simulink model "ScriptDemo"  (R2022b)
settings: configuration reference "TmVcThermal_Configuration_sub" (kept outside this file)
undefined symbols (not defined in the file): aaaa, bbbb, cTmComprCtrl_D_u8HvacFlowTable_db, cTmComprCtrl_D_u8HvacFlowTable_sw, cTmComprCtrl_n_i16ChillCmpIMax, cTmComprCtrl_n_i16ChillCmpIMin, cTmComprCtrl_n_i16ChillCmpIMin666, cTmComprCtrl_n_i16ChillCmpPMax, cTmComprCtrl_n_i16ChillCmpPMin, cTmComprCtrl_n_i16CmpChillCoolRpmKiMax, cTmComprCtrl_n_i16CmpChillCoolRpmKiMin, cTmComprCtrl_n_i16CmpChillCoolRpmKpMax, cTmComprCtrl_n_i16CmpChillCoolRpmKpMin, cTmComprCtrl_n_i16CmpCoolRpmKiMax, cTmComprCtrl_n_i16CmpCoolRpmKiMin, cTmComprCtrl_n_i16CmpCoolRpmKpMax, cTmComprCtrl_n_i16CmpCoolRpmKpMin, cTmComprCtrl_n_i16SM4CmpHeatKiMax, cTmComprCtrl_n_i16SM4CmpHeatKiMin, cTmComprCtrl_n_i16SM4CmpHeatKpMax, cTmComprCtrl_n_i16SM4CmpHeatKpMin, cTmComprCtrl_n_i16SM5CmpHeatKiMax, cTmComprCtrl_n_i16SM5CmpHeatKiMin, cTmComprCtrl_n_i16SM5CmpHeatKpMax, cTmComprCtrl_n_i16SM5CmpHeatKpMin, cTmComprCtrl_n_i16SM6CmpHeatKiMax, cTmComprCtrl_n_i16SM6CmpHeatKiMin, cTmComprCtrl_n_i16SM6CmpHeatKpMax, cTmComprCtrl_n_i16SM6CmpHeatKpMin, cTmComprCtrl_n_u16CmpMaxSpdFanFltLimt, cTmComprCtrl_n_u16CmpMaxSpdLoSidePFltLimt, cTmComprCtrl_n_u16CmpMaxSpdSensorFltLimt, cTmComprCtrl_n_u16CompMinRpm, cTmComprCtrl_n_u16CompRpmIncThres, cTmComprCtrl_t_u16BattCooltFFPeriod, cTmComprCtrl_t_u16BattCooltPIPeriod, cTmComprCtrl_t_u16CmpCoolFFPeriod, cTmComprCtrl_t_u16CmpCoolPIPeriod, cTmComprCtrl_t_u16CoolCmpChillFFPeriod, cTmComprCtrl_t_u16CoolCmpChillPIPeriod, cTmComprCtrl_t_u16SM4CmpHeatFFPeriod, cTmComprCtrl_t_u16SM4CmpHeatPIPeriod, cTmComprCtrl_t_u16SM5CmpHeatFFPeriod, cTmComprCtrl_t_u16SM5CmpHeatPIPeriod, cTmComprCtrl_t_u16SM6CmpHeatFFPeriod, cTmComprCtrl_t_u16SM6CmpHeatPIPeriod, cTmComprCtrl_Te_EvapClearInteg, cTmComprCtrl_Te_i16HpReqTempSaturoffset, cTmComprCtrl_Te_i16SatLpReplaceDiff, cTmComprCtrl_Te_i16SM3BatDiffStartEvapDecOffset, cTmComprCtrl_Te_i16SM3EvapLo, cTmComprCtrl_Te_i16SM3TBatDiffEntEvapDecOffset, cTmComprCtrl_Te_i16SM3TBatDiffEntEvapDecOffsetQuit, cTmComprCtrl_Te_s32ErrCmpChillPIContinueCoolH, cTmComprCtrl_Te_s32ErrCmpChillPIContinueCoolL, cTmComprCtrl_Te_s32ErrCmpPIContinueChillH, cTmComprCtrl_Te_s32ErrCmpPIContinueChillL, cTmComprCtrl_Te_s32ErrCmpPIContinueCoolH, cTmComprCtrl_Te_s32ErrCmpPIContinueCoolL, cTmComprCtrl_Te_s32ErrCmpPIContinueHeatH ... (+398)
libraries: simulink x782, PCMULib x640, simulink_need_slupdate x4
(part 2 of 41)

== system ScriptDemo/Change/changeModSizeGcs/Before ==
  rTmComprCtrl_n_u16CompRpmReqModeOut : Inport  OutDataTypeStr=uint16
  sTmDiag_D_u8CmprDischrgTFltSt : Inport  Port=2  OutDataTypeStr=uint8
  sTmDiag_D_u8FanFltSt : Inport  Port=3  OutDataTypeStr=uint8
  sTmDiag_D_u8HiSidePFltSt : Inport  Port=4  OutDataTypeStr=uint8
  sTmDiag_D_u8OutrCondOutTFltSt : Inport  Port=5  OutDataTypeStr=uint8
  sTmSigProces_Te_s32TAmb : Inport  Port=6  OutDataTypeStr=single
  sTmIn_n_s32ElacCmprActl : Inport  Port=7  OutDataTypeStr=single
  sTmIn_v_s32VehSpdLgt : Inport  Port=8  OutDataTypeStr=single
  sTmRefriModeMgr_D_u8HPCurMode : Inport  Port=9  OutDataTypeStr=uint8
  sTmRefriModeMgr_D_u8HpFmCmd : Inport  Port=10  OutDataTypeStr=uint8
  sTmSigProces_Pw_i16ReqPwrForHeat : Inport  Port=11  OutDataTypeStr=int16
  sTmSigProces_Te_s32CompDischarge : Inport  Port=12  OutDataTypeStr=single
  sTmSigProces_md_u16BlwCool : Inport  Port=13  OutDataTypeStr=uint16
  sTmSigProces_p_u16PHighSide : Inport  Port=14  OutDataTypeStr=uint16
  sTmSigProces_p_u16PLowSide : Inport  Port=15  OutDataTypeStr=uint16
  sTmIn_D_u8HeatPump : Inport  Port=16  OutDataTypeStr=uint8
  sTmIn_D_u8ElecDriveline : Inport  Port=17
  sTmSigProces_D_u8CarChrgMode : Inport  Port=18  OutDataTypeStr=uint8
  sTmSigProces_md_u16BlwHeat : Inport  Port=19  OutDataTypeStr=uint16
  sTmDiag_D_u8LoSidePFltSt : Inport  Port=20  OutDataTypeStr=uint8
  xTmComprCtrl_B_CompOnReqCompOn : Inport  Port=21  OutDataTypeStr=boolean
  rTmComprCtrl_n_u16CompRpmReqModeOut1 : Inport  Port=22  OutDataTypeStr=uint16
  sTmDiag_D_u8CmprDischrgTFltSt1 : Inport  Port=23  OutDataTypeStr=uint8
  sTmDiag_D_u8FanFltSt1 : Inport  Port=24  OutDataTypeStr=uint8
  sTmDiag_D_u8HiSidePFltSt1 : Inport  Port=25  OutDataTypeStr=uint8
  sTmDiag_D_u8OutrCondOutTFltSt1 : Inport  Port=26  OutDataTypeStr=uint8
  sTmSigProces_Te_s32TAmb1 : Inport  Port=27  OutDataTypeStr=single
  sTmIn_n_s32ElacCmprActl1 : Inport  Port=28  OutDataTypeStr=single
  sTmIn_v_s32VehSpdLgt1 : Inport  Port=29  OutDataTypeStr=single
  sTmRefriModeMgr_D_u8HPCurMode1 : Inport  Port=30  OutDataTypeStr=uint8
  sTmRefriModeMgr_D_u8HpFmCmd1 : Inport  Port=31  OutDataTypeStr=uint8
  sTmSigProces_Pw_i16ReqPwrForHeat1 : Inport  Port=32  OutDataTypeStr=int16
  sTmSigProces_Te_s32CompDischarge1 : Inport  Port=33  OutDataTypeStr=single
  rTmComprCtrl_n_u16CompRpmReqModeOut2 : Inport  Port=34  OutDataTypeStr=uint16
  sTmDiag_D_u8CmprDischrgTFltSt2 : Inport  Port=35  OutDataTypeStr=uint8
  sTmDiag_D_u8FanFltSt2 : Inport  Port=36  OutDataTypeStr=uint8
  sTmDiag_D_u8HiSidePFltSt2 : Inport  Port=37  OutDataTypeStr=uint8
  sTmDiag_D_u8OutrCondOutTFltSt2 : Inport  Port=38  OutDataTypeStr=uint8
  sTmSigProces_Te_s32TAmb2 : Inport  Port=39  OutDataTypeStr=single
  sTmIn_n_s32ElacCmprActl2 : Inport  Port=40  OutDataTypeStr=single
  sTmIn_v_s32VehSpdLgt2 : Inport  Port=41  OutDataTypeStr=single
  sTmRefriModeMgr_D_u8HPCurMode2 : Inport  Port=42  OutDataTypeStr=uint8
  sTmRefriModeMgr_D_u8HpFmCmd2 : Inport  Port=43  OutDataTypeStr=uint8
  sTmSigProces_Pw_i16ReqPwrForHeat2 : Inport  Port=44  OutDataTypeStr=int16
  sTmSigProces_Te_s32CompDischarge2 : Inport  Port=45  OutDataTypeStr=single
  sTmSigProces_md_u16BlwCool2 : Inport  Port=46  OutDataTypeStr=uint16
  sTmSigProces_p_u16PHighSide2 : Inport  Port=47  OutDataTypeStr=uint16
  sTmSigProces_p_u16PLowSide2 : Inport  Port=48  OutDataTypeStr=uint16
  sTmIn_D_u8HeatPump2 : Inport  Port=49  OutDataTypeStr=uint8
  sTmIn_D_u8ElecDriveline2 : Inport  Port=50
  sTmSigProces_D_u8CarChrgMode2 : Inport  Port=51  OutDataTypeStr=uint8
  sTmSigProces_md_u16BlwHeat2 : Inport  Port=52  OutDataTypeStr=uint16
  sTmDiag_D_u8LoSidePFltSt2 : Inport  Port=53  OutDataTypeStr=uint8
  xTmComprCtrl_B_CompOnReqCompOn2 : Inport  Port=54  OutDataTypeStr=boolean
  rTmComprCtrl_n_u16CompRpmReqModeOut3 : Inport  Port=55  OutDataTypeStr=uint16
  sTmDiag_D_u8CmprDischrgTFltSt3 : Inport  Port=56  OutDataTypeStr=uint8
  sTmDiag_D_u8FanFltSt3 : Inport  Port=57  OutDataTypeStr=uint8
  sTmDiag_D_u8HiSidePFltSt3 : Inport  Port=58  OutDataTypeStr=uint8
  sTmDiag_D_u8OutrCondOutTFltSt3 : Inport  Port=59  OutDataTypeStr=uint8
  sTmSigProces_Te_s32TAmb3 : Inport  Port=60  OutDataTypeStr=single
  sTmIn_n_s32ElacCmprActl3 : Inport  Port=61  OutDataTypeStr=single
  sTmIn_v_s32VehSpdLgt3 : Inport  Port=62  OutDataTypeStr=single
  sTmRefriModeMgr_D_u8HPCurMode3 : Inport  Port=63  OutDataTypeStr=uint8
  sTmRefriModeMgr_D_u8HpFmCmd3 : Inport  Port=64  OutDataTypeStr=uint8
  sTmSigProces_Pw_i16ReqPwrForHeat3 : Inport  Port=65  OutDataTypeStr=int16
  sTmSigProces_Te_s32CompDischarge3 : Inport  Port=66  OutDataTypeStr=single
  sTmSigProces_md_u16BlwCool3 : Inport  Port=67  OutDataTypeStr=uint16
  sTmSigProces_p_u16PHighSide3 : Inport  Port=68  OutDataTypeStr=uint16
  sTmSigProces_p_u16PLowSide3 : Inport  Port=69  OutDataTypeStr=uint16
  sTmIn_D_u8HeatPump3 : Inport  Port=70  OutDataTypeStr=uint8
  sTmIn_D_u8ElecDriveline3 : Inport  Port=71
  sTmSigProces_D_u8CarChrgMode3 : Inport  Port=72  OutDataTypeStr=uint8
  sTmSigProces_md_u16BlwHeat3 : Inport  Port=73  OutDataTypeStr=uint16
  sTmDiag_D_u8LoSidePFltSt3 : Inport  Port=74  OutDataTypeStr=uint8
  xTmComprCtrl_B_CompOnReqCompOn3 : Inport  Port=75  OutDataTypeStr=boolean
  Subsystem : Subsystem
  Subsystem1 : Subsystem
  Subsystem2 : Subsystem
  Subsystem3 : Subsystem
  rTmComprCtrl_n_u16CompRpmReqFilter : Outport  OutDataTypeStr=uint16
  xTmComprCtrl_B_KeepRpm : Outport  Port=2  OutDataTypeStr=boolean
  xFilter_B_ComprStop : Outport  Port=3  OutDataTypeStr=boolean
  sFilter_n_u16CompMaxRpm : Outport  Port=4  OutDataTypeStr=uint16
  rFilter_p_u16AcHiSideHiCut : Outport  Port=5  OutDataTypeStr=uint16
  rFilter_p_u16CmpLimitNormalP : Outport  Port=6  OutDataTypeStr=uint16
  rFilter_p_u16CmpLimitLowP : Outport  Port=7  OutDataTypeStr=uint16
  rFilter_p_u16CmpLimitMidP : Outport  Port=8  OutDataTypeStr=uint16
  rFilter_p_u16CmpLimitShutDownP : Outport  Port=9  OutDataTypeStr=uint16
  xTmComprCtrl_B_ReduceRpm : Outport  Port=10  OutDataTypeStr=boolean
  rTmComprCtrl_n_u16CompRpmReqFilter1 : Outport  Port=11  OutDataTypeStr=uint16
  xTmComprCtrl_B_KeepRpm1 : Outport  Port=12  OutDataTypeStr=boolean
  xFilter_B_ComprStop1 : Outport  Port=13  OutDataTypeStr=boolean
  sFilter_n_u16CompMaxRpm1 : Outport  Port=14  OutDataTypeStr=uint16
  rFilter_p_u16AcHiSideHiCut1 : Outport  Port=15  OutDataTypeStr=uint16
  rFilter_p_u16CmpLimitNormalP1 : Outport  Port=16  OutDataTypeStr=uint16
  rFilter_p_u16CmpLimitLowP1 : Outport  Port=17  OutDataTypeStr=uint16
  rFilter_p_u16CmpLimitMidP1 : Outport  Port=18  OutDataTypeStr=uint16
  rFilter_p_u16CmpLimitShutDownP1 : Outport  Port=19  OutDataTypeStr=uint16
  xTmComprCtrl_B_ReduceRpm1 : Outport  Port=20  OutDataTypeStr=boolean
  rTmComprCtrl_n_u16CompRpmReqFilter2 : Outport  Port=21  OutDataTypeStr=uint16
  xTmComprCtrl_B_KeepRpm2 : Outport  Port=22  OutDataTypeStr=boolean
  xFilter_B_ComprStop2 : Outport  Port=23  OutDataTypeStr=boolean
  sFilter_n_u16CompMaxRpm2 : Outport  Port=24  OutDataTypeStr=uint16
  rFilter_p_u16AcHiSideHiCut2 : Outport  Port=25  OutDataTypeStr=uint16
  rFilter_p_u16CmpLimitNormalP2 : Outport  Port=26  OutDataTypeStr=uint16
  rFilter_p_u16CmpLimitLowP2 : Outport  Port=27  OutDataTypeStr=uint16
  rFilter_p_u16CmpLimitMidP2 : Outport  Port=28  OutDataTypeStr=uint16
  rFilter_p_u16CmpLimitShutDownP2 : Outport  Port=29  OutDataTypeStr=uint16
  xTmComprCtrl_B_ReduceRpm2 : Outport  Port=30  OutDataTypeStr=boolean
  rTmComprCtrl_n_u16CompRpmReqFilter3 : Outport  Port=31  OutDataTypeStr=uint16
  xTmComprCtrl_B_KeepRpm3 : Outport  Port=32  OutDataTypeStr=boolean
  xFilter_B_ComprStop3 : Outport  Port=33  OutDataTypeStr=boolean
  sFilter_n_u16CompMaxRpm3 : Outport  Port=34  OutDataTypeStr=uint16
  rFilter_p_u16AcHiSideHiCut3 : Outport  Port=35  OutDataTypeStr=uint16
  rFilter_p_u16CmpLimitNormalP3 : Outport  Port=36  OutDataTypeStr=uint16
  rFilter_p_u16CmpLimitLowP3 : Outport  Port=37  OutDataTypeStr=uint16
  rFilter_p_u16CmpLimitMidP3 : Outport  Port=38  OutDataTypeStr=uint16
  rFilter_p_u16CmpLimitShutDownP3 : Outport  Port=39  OutDataTypeStr=uint16
  xTmComprCtrl_B_ReduceRpm3 : Outport  Port=40  OutDataTypeStr=boolean
  wires:
  Subsystem/7(rFilter_p_u16CmpLimitLowP) -> rFilter_p_u16CmpLimitLowP/1
  Subsystem/2(xTmComprCtrl_B_KeepRpm) -> xTmComprCtrl_B_KeepRpm/1
  Subsystem/8(rFilter_p_u16CmpLimitMidP) -> rFilter_p_u16CmpLimitMidP/1
  Subsystem/9(rFilter_p_u16CmpLimitShutDownP) -> rFilter_p_u16CmpLimitShutDownP/1
  Subsystem/6(rFilter_p_u16CmpLimitNormalP) -> rFilter_p_u16CmpLimitNormalP/1
  Subsystem/5(rFilter_p_u16AcHiSideHiCut) -> rFilter_p_u16AcHiSideHiCut/1
  Subsystem/3(xFilter_B_ComprStop) -> xFilter_B_ComprStop/1
  Subsystem/4(sFilter_n_u16CompMaxRpm) -> sFilter_n_u16CompMaxRpm/1
  sTmSigProces_D_u8CarChrgMode/1 -> Subsystem/18(sTmSigProces_D_u8CarChrgMode)
  sTmSigProces_md_u16BlwHeat/1 -> Subsystem/19(sTmSigProces_md_u16BlwHeat)
  sTmSigProces_p_u16PLowSide/1 -> Subsystem/15(sTmSigProces_p_u16PLowSide)
  sTmIn_D_u8HeatPump/1 -> Subsystem/16(sTmIn_D_u8HeatPump)
  sTmIn_D_u8ElecDriveline/1 -> Subsystem/17(sTmIn_D_u8ElecDriveline)
  sTmDiag_D_u8LoSidePFltSt/1 -> Subsystem/20(sTmDiag_D_u8LoSidePFltSt)
  sTmSigProces_Te_s32TAmb/1 -> Subsystem/6(sTmSigProces_Te_s32TAmb)
  sTmIn_n_s32ElacCmprActl/1 -> Subsystem/7(sTmIn_n_s32ElacCmprActl)
  sTmSigProces_Te_s32CompDischarge/1 -> Subsystem/12(sTmSigProces_Te_s32CompDischarge)
  sTmRefriModeMgr_D_u8HPCurMode/1 -> Subsystem/9(sTmRefriModeMgr_D_u8HPCurMode)
  sTmSigProces_Pw_i16ReqPwrForHeat/1 -> Subsystem/11(sTmSigProces_Pw_i16ReqPwrForHeat)
  sTmRefriModeMgr_D_u8HpFmCmd/1 -> Subsystem/10(sTmRefriModeMgr_D_u8HpFmCmd)
  sTmDiag_D_u8OutrCondOutTFltSt/1 -> Subsystem/5(sTmDiag_D_u8OutrCondOutTFltSt)
  sTmIn_v_s32VehSpdLgt/1 -> Subsystem/8(sTmIn_v_s32VehSpdLgt)
  sTmSigProces_md_u16BlwCool/1 -> Subsystem/13(sTmSigProces_md_u16BlwCool)
  sTmDiag_D_u8FanFltSt/1 -> Subsystem/3(sTmDiag_D_u8FanFltSt)
  sTmDiag_D_u8HiSidePFltSt/1 -> Subsystem/4(sTmDiag_D_u8HiSidePFltSt)
  xTmComprCtrl_B_CompOnReqCompOn/1 -> Subsystem/21(xTmComprCtrl_B_CompOnReqCompOn)
  sTmDiag_D_u8CmprDischrgTFltSt/1 -> Subsystem/2(sTmDiag_D_u8CmprDischrgTFltSt)
  rTmComprCtrl_n_u16CompRpmReqModeOut/1 -> Subsystem/1(rTmComprCtrl_n_u16CompRpmReqModeOut)
  Subsystem/1(rTmComprCtrl_n_u16CompRpmReqFilter) -> rTmComprCtrl_n_u16CompRpmReqFilter/1
  sTmSigProces_p_u16PHighSide/1 -> Subsystem/14(sTmSigProces_p_u16PHighSide)
  Subsystem/10(xTmComprCtrl_B_ReduceRpm) -> xTmComprCtrl_B_ReduceRpm/1
  Subsystem1/1(rTmComprCtrl_n_u16CompRpmReqFilter) -> rTmComprCtrl_n_u16CompRpmReqFilter1/1
  Subsystem1/10(xTmComprCtrl_B_ReduceRpm) -> xTmComprCtrl_B_ReduceRpm1/1
  rTmComprCtrl_n_u16CompRpmReqModeOut1/1 -> Subsystem1/1(rTmComprCtrl_n_u16CompRpmReqModeOut)
  sTmDiag_D_u8HiSidePFltSt1/1 -> Subsystem1/4(sTmDiag_D_u8HiSidePFltSt)
  sTmDiag_D_u8FanFltSt1/1 -> Subsystem1/3(sTmDiag_D_u8FanFltSt)
  Subsystem1/2(xTmComprCtrl_B_KeepRpm) -> xTmComprCtrl_B_KeepRpm1/1
  Subsystem1/7(rFilter_p_u16CmpLimitLowP) -> rFilter_p_u16CmpLimitLowP1/1
  sTmDiag_D_u8OutrCondOutTFltSt1/1 -> Subsystem1/5(sTmDiag_D_u8OutrCondOutTFltSt)
  sTmSigProces_Pw_i16ReqPwrForHeat1/1 -> Subsystem1/11(sTmSigProces_Pw_i16ReqPwrForHeat)
  sTmRefriModeMgr_D_u8HpFmCmd1/1 -> Subsystem1/10(sTmRefriModeMgr_D_u8HpFmCmd)
  sTmSigProces_Te_s32CompDischarge1/1 -> Subsystem1/12(sTmSigProces_Te_s32CompDischarge)
  sTmIn_n_s32ElacCmprActl1/1 -> Subsystem1/7(sTmIn_n_s32ElacCmprActl)
  sTmRefriModeMgr_D_u8HPCurMode1/1 -> Subsystem1/9(sTmRefriModeMgr_D_u8HPCurMode)
  sTmIn_v_s32VehSpdLgt1/1 -> Subsystem1/8(sTmIn_v_s32VehSpdLgt)
  Subsystem1/3(xFilter_B_ComprStop) -> xFilter_B_ComprStop1/1
  sTmSigProces_Te_s32TAmb1/1 -> Subsystem1/6(sTmSigProces_Te_s32TAmb)
  Subsystem1/5(rFilter_p_u16AcHiSideHiCut) -> rFilter_p_u16AcHiSideHiCut1/1
  sTmDiag_D_u8CmprDischrgTFltSt1/1 -> Subsystem1/2(sTmDiag_D_u8CmprDischrgTFltSt)
  Subsystem1/6(rFilter_p_u16CmpLimitNormalP) -> rFilter_p_u16CmpLimitNormalP1/1
  Subsystem1/4(sFilter_n_u16CompMaxRpm) -> sFilter_n_u16CompMaxRpm1/1
  Subsystem1/9(rFilter_p_u16CmpLimitShutDownP) -> rFilter_p_u16CmpLimitShutDownP1/1
  Subsystem1/8(rFilter_p_u16CmpLimitMidP) -> rFilter_p_u16CmpLimitMidP1/1
  Subsystem2/1(rTmComprCtrl_n_u16CompRpmReqFilter) -> rTmComprCtrl_n_u16CompRpmReqFilter2/1
  Subsystem2/10(xTmComprCtrl_B_ReduceRpm) -> xTmComprCtrl_B_ReduceRpm2/1
  sTmSigProces_p_u16PHighSide2/1 -> Subsystem2/14(sTmSigProces_p_u16PHighSide)
  rTmComprCtrl_n_u16CompRpmReqModeOut2/1 -> Subsystem2/1(rTmComprCtrl_n_u16CompRpmReqModeOut)
  sTmDiag_D_u8HiSidePFltSt2/1 -> Subsystem2/4(sTmDiag_D_u8HiSidePFltSt)
  sTmDiag_D_u8FanFltSt2/1 -> Subsystem2/3(sTmDiag_D_u8FanFltSt)
  Subsystem2/2(xTmComprCtrl_B_KeepRpm) -> xTmComprCtrl_B_KeepRpm2/1
  Subsystem2/7(rFilter_p_u16CmpLimitLowP) -> rFilter_p_u16CmpLimitLowP2/1
  sTmSigProces_md_u16BlwCool2/1 -> Subsystem2/13(sTmSigProces_md_u16BlwCool)
  sTmDiag_D_u8LoSidePFltSt2/1 -> Subsystem2/20(sTmDiag_D_u8LoSidePFltSt)
  sTmDiag_D_u8OutrCondOutTFltSt2/1 -> Subsystem2/5(sTmDiag_D_u8OutrCondOutTFltSt)
  xTmComprCtrl_B_CompOnReqCompOn2/1 -> Subsystem2/21(xTmComprCtrl_B_CompOnReqCompOn)
  sTmSigProces_Pw_i16ReqPwrForHeat2/1 -> Subsystem2/11(sTmSigProces_Pw_i16ReqPwrForHeat)
  sTmRefriModeMgr_D_u8HpFmCmd2/1 -> Subsystem2/10(sTmRefriModeMgr_D_u8HpFmCmd)
  sTmSigProces_Te_s32CompDischarge2/1 -> Subsystem2/12(sTmSigProces_Te_s32CompDischarge)
  sTmIn_n_s32ElacCmprActl2/1 -> Subsystem2/7(sTmIn_n_s32ElacCmprActl)
  sTmIn_D_u8HeatPump2/1 -> Subsystem2/16(sTmIn_D_u8HeatPump)
  sTmSigProces_p_u16PLowSide2/1 -> Subsystem2/15(sTmSigProces_p_u16PLowSide)
  sTmRefriModeMgr_D_u8HPCurMode2/1 -> Subsystem2/9(sTmRefriModeMgr_D_u8HPCurMode)
  sTmIn_v_s32VehSpdLgt2/1 -> Subsystem2/8(sTmIn_v_s32VehSpdLgt)
  sTmSigProces_D_u8CarChrgMode2/1 -> Subsystem2/18(sTmSigProces_D_u8CarChrgMode)
  Subsystem2/3(xFilter_B_ComprStop) -> xFilter_B_ComprStop2/1
  sTmSigProces_Te_s32TAmb2/1 -> Subsystem2/6(sTmSigProces_Te_s32TAmb)
  sTmSigProces_md_u16BlwHeat2/1 -> Subsystem2/19(sTmSigProces_md_u16BlwHeat)
  Subsystem2/5(rFilter_p_u16AcHiSideHiCut) -> rFilter_p_u16AcHiSideHiCut2/1
  sTmDiag_D_u8CmprDischrgTFltSt2/1 -> Subsystem2/2(sTmDiag_D_u8CmprDischrgTFltSt)
  Subsystem2/6(rFilter_p_u16CmpLimitNormalP) -> rFilter_p_u16CmpLimitNormalP2/1
  Subsystem2/4(sFilter_n_u16CompMaxRpm) -> sFilter_n_u16CompMaxRpm2/1
  sTmIn_D_u8ElecDriveline2/1 -> Subsystem2/17(sTmIn_D_u8ElecDriveline)
  Subsystem2/9(rFilter_p_u16CmpLimitShutDownP) -> rFilter_p_u16CmpLimitShutDownP2/1
  Subsystem2/8(rFilter_p_u16CmpLimitMidP) -> rFilter_p_u16CmpLimitMidP2/1
  Subsystem3/1(rTmComprCtrl_n_u16CompRpmReqFilter) -> rTmComprCtrl_n_u16CompRpmReqFilter3/1
  Subsystem3/10(xTmComprCtrl_B_ReduceRpm) -> xTmComprCtrl_B_ReduceRpm3/1
  sTmSigProces_p_u16PHighSide3/1 -> Subsystem3/14(sTmSigProces_p_u16PHighSide)
  rTmComprCtrl_n_u16CompRpmReqModeOut3/1 -> Subsystem3/1(rTmComprCtrl_n_u16CompRpmReqModeOut)
  sTmDiag_D_u8HiSidePFltSt3/1 -> Subsystem3/4(sTmDiag_D_u8HiSidePFltSt)
  sTmDiag_D_u8FanFltSt3/1 -> Subsystem3/3(sTmDiag_D_u8FanFltSt)
  Subsystem3/2(xTmComprCtrl_B_KeepRpm) -> xTmComprCtrl_B_KeepRpm3/1
  Subsystem3/7(rFilter_p_u16CmpLimitLowP) -> rFilter_p_u16CmpLimitLowP3/1
  sTmSigProces_md_u16BlwCool3/1 -> Subsystem3/13(sTmSigProces_md_u16BlwCool)
  sTmDiag_D_u8LoSidePFltSt3/1 -> Subsystem3/20(sTmDiag_D_u8LoSidePFltSt)
  sTmDiag_D_u8OutrCondOutTFltSt3/1 -> Subsystem3/5(sTmDiag_D_u8OutrCondOutTFltSt)
  xTmComprCtrl_B_CompOnReqCompOn3/1 -> Subsystem3/21(xTmComprCtrl_B_CompOnReqCompOn)
  sTmSigProces_Pw_i16ReqPwrForHeat3/1 -> Subsystem3/11(sTmSigProces_Pw_i16ReqPwrForHeat)
  sTmRefriModeMgr_D_u8HpFmCmd3/1 -> Subsystem3/10(sTmRefriModeMgr_D_u8HpFmCmd)
  sTmSigProces_Te_s32CompDischarge3/1 -> Subsystem3/12(sTmSigProces_Te_s32CompDischarge)
  sTmIn_n_s32ElacCmprActl3/1 -> Subsystem3/7(sTmIn_n_s32ElacCmprActl)
  sTmIn_D_u8HeatPump3/1 -> Subsystem3/16(sTmIn_D_u8HeatPump)
  sTmSigProces_p_u16PLowSide3/1 -> Subsystem3/15(sTmSigProces_p_u16PLowSide)
  sTmRefriModeMgr_D_u8HPCurMode3/1 -> Subsystem3/9(sTmRefriModeMgr_D_u8HPCurMode)
  sTmIn_v_s32VehSpdLgt3/1 -> Subsystem3/8(sTmIn_v_s32VehSpdLgt)
  sTmSigProces_D_u8CarChrgMode3/1 -> Subsystem3/18(sTmSigProces_D_u8CarChrgMode)
  Subsystem3/3(xFilter_B_ComprStop) -> xFilter_B_ComprStop3/1
  sTmSigProces_Te_s32TAmb3/1 -> Subsystem3/6(sTmSigProces_Te_s32TAmb)
  sTmSigProces_md_u16BlwHeat3/1 -> Subsystem3/19(sTmSigProces_md_u16BlwHeat)
  Subsystem3/5(rFilter_p_u16AcHiSideHiCut) -> rFilter_p_u16AcHiSideHiCut3/1
  sTmDiag_D_u8CmprDischrgTFltSt3/1 -> Subsystem3/2(sTmDiag_D_u8CmprDischrgTFltSt)
  Subsystem3/6(rFilter_p_u16CmpLimitNormalP) -> rFilter_p_u16CmpLimitNormalP3/1
  Subsystem3/4(sFilter_n_u16CompMaxRpm) -> sFilter_n_u16CompMaxRpm3/1
  sTmIn_D_u8ElecDriveline3/1 -> Subsystem3/17(sTmIn_D_u8ElecDriveline)
  Subsystem3/9(rFilter_p_u16CmpLimitShutDownP) -> rFilter_p_u16CmpLimitShutDownP3/1
  Subsystem3/8(rFilter_p_u16CmpLimitMidP) -> rFilter_p_u16CmpLimitMidP3/1

== system ScriptDemo/Change/changeModSizeGcs/Before1 ==
  rTmComprCtrl_n_u16CompRpmReqModeOut : Inport  OutDataTypeStr=uint16
  sTmDiag_D_u8CmprDischrgTFltSt : Inport  Port=2  OutDataTypeStr=uint8
  sTmDiag_D_u8FanFltSt : Inport  Port=3  OutDataTypeStr=uint8
  sTmDiag_D_u8HiSidePFltSt : Inport  Port=4  OutDataTypeStr=uint8
  sTmDiag_D_u8OutrCondOutTFltSt : Inport  Port=5  OutDataTypeStr=uint8
  sTmSigProces_Te_s32TAmb : Inport  Port=6  OutDataTypeStr=single
  sTmIn_n_s32ElacCmprActl : Inport  Port=7  OutDataTypeStr=single
  sTmIn_v_s32VehSpdLgt : Inport  Port=8  OutDataTypeStr=single
  sTmRefriModeMgr_D_u8HPCurMode : Inport  Port=9  OutDataTypeStr=uint8
  sTmRefriModeMgr_D_u8HpFmCmd : Inport  Port=10  OutDataTypeStr=uint8
  sTmSigProces_Pw_i16ReqPwrForHeat : Inport  Port=11  OutDataTypeStr=int16
  sTmSigProces_Te_s32CompDischarge : Inport  Port=12  OutDataTypeStr=single
  sTmSigProces_md_u16BlwCool : Inport  Port=13  OutDataTypeStr=uint16
  sTmSigProces_p_u16PHighSide : Inport  Port=14  OutDataTypeStr=uint16
  sTmSigProces_p_u16PLowSide : Inport  Port=15  OutDataTypeStr=uint16
  sTmIn_D_u8HeatPump : Inport  Port=16  OutDataTypeStr=uint8
  sTmIn_D_u8ElecDriveline : Inport  Port=17
  sTmSigProces_D_u8CarChrgMode : Inport  Port=18  OutDataTypeStr=uint8
  sTmSigProces_md_u16BlwHeat : Inport  Port=19  OutDataTypeStr=uint16
  sTmDiag_D_u8LoSidePFltSt : Inport  Port=20  OutDataTypeStr=uint8
  xTmComprCtrl_B_CompOnReqCompOn : Inport  Port=21  OutDataTypeStr=boolean
  rTmComprCtrl_n_u16CompRpmReqModeOut1 : Inport  Port=22  OutDataTypeStr=uint16
  sTmDiag_D_u8CmprDischrgTFltSt1 : Inport  Port=23  OutDataTypeStr=uint8
  sTmDiag_D_u8FanFltSt1 : Inport  Port=24  OutDataTypeStr=uint8
  sTmDiag_D_u8HiSidePFltSt1 : Inport  Port=25  OutDataTypeStr=uint8
  sTmDiag_D_u8OutrCondOutTFltSt1 : Inport  Port=26  OutDataTypeStr=uint8
  sTmSigProces_Te_s32TAmb1 : Inport  Port=27  OutDataTypeStr=single
  sTmIn_n_s32ElacCmprActl1 : Inport  Port=28  OutDataTypeStr=single
  sTmIn_v_s32VehSpdLgt1 : Inport  Port=29  OutDataTypeStr=single
  sTmRefriModeMgr_D_u8HPCurMode1 : Inport  Port=30  OutDataTypeStr=uint8
  sTmRefriModeMgr_D_u8HpFmCmd1 : Inport  Port=31  OutDataTypeStr=uint8
  sTmSigProces_Pw_i16ReqPwrForHeat1 : Inport  Port=32  OutDataTypeStr=int16
  sTmSigProces_Te_s32CompDischarge1 : Inport  Port=33  OutDataTypeStr=single
  rTmComprCtrl_n_u16CompRpmReqModeOut2 : Inport  Port=34  OutDataTypeStr=uint16
  sTmDiag_D_u8CmprDischrgTFltSt2 : Inport  Port=35  OutDataTypeStr=uint8
  sTmDiag_D_u8FanFltSt2 : Inport  Port=36  OutDataTypeStr=uint8
  sTmDiag_D_u8HiSidePFltSt2 : Inport  Port=37  OutDataTypeStr=uint8
  sTmDiag_D_u8OutrCondOutTFltSt2 : Inport  Port=38  OutDataTypeStr=uint8
  sTmSigProces_Te_s32TAmb2 : Inport  Port=39  OutDataTypeStr=single
  sTmIn_n_s32ElacCmprActl2 : Inport  Port=40  OutDataTypeStr=single
  sTmIn_v_s32VehSpdLgt2 : Inport  Port=41  OutDataTypeStr=single
  sTmRefriModeMgr_D_u8HPCurMode2 : Inport  Port=42  OutDataTypeStr=uint8
  sTmRefriModeMgr_D_u8HpFmCmd2 : Inport  Port=43  OutDataTypeStr=uint8
  sTmSigProces_Pw_i16ReqPwrForHeat2 : Inport  Port=44  OutDataTypeStr=int16
  sTmSigProces_Te_s32CompDischarge2 : Inport  Port=45  OutDataTypeStr=single
  sTmSigProces_md_u16BlwCool2 : Inport  Port=46  OutDataTypeStr=uint16
  sTmSigProces_p_u16PHighSide2 : Inport  Port=47  OutDataTypeStr=uint16
  sTmSigProces_p_u16PLowSide2 : Inport  Port=48  OutDataTypeStr=uint16
  sTmIn_D_u8HeatPump2 : Inport  Port=49  OutDataTypeStr=uint8
  sTmIn_D_u8ElecDriveline2 : Inport  Port=50
  sTmSigProces_D_u8CarChrgMode2 : Inport  Port=51  OutDataTypeStr=uint8
  sTmSigProces_md_u16BlwHeat2 : Inport  Port=52  OutDataTypeStr=uint16
  sTmDiag_D_u8LoSidePFltSt2 : Inport  Port=53  OutDataTypeStr=uint8
  xTmComprCtrl_B_CompOnReqCompOn2 : Inport  Port=54  OutDataTypeStr=boolean
  rTmComprCtrl_n_u16CompRpmReqModeOut3 : Inport  Port=55  OutDataTypeStr=uint16
  sTmDiag_D_u8CmprDischrgTFltSt3 : Inport  Port=56  OutDataTypeStr=uint8
  sTmDiag_D_u8FanFltSt3 : Inport  Port=57  OutDataTypeStr=uint8
  sTmDiag_D_u8HiSidePFltSt3 : Inport  Port=58  OutDataTypeStr=uint8
  sTmDiag_D_u8OutrCondOutTFltSt3 : Inport  Port=59  OutDataTypeStr=uint8
  sTmSigProces_Te_s32TAmb3 : Inport  Port=60  OutDataTypeStr=single
  sTmIn_n_s32ElacCmprActl3 : Inport  Port=61  OutDataTypeStr=single
  sTmIn_v_s32VehSpdLgt3 : Inport  Port=62  OutDataTypeStr=single
  sTmRefriModeMgr_D_u8HPCurMode3 : Inport  Port=63  OutDataTypeStr=uint8
  sTmRefriModeMgr_D_u8HpFmCmd3 : Inport  Port=64  OutDataTypeStr=uint8
  sTmSigProces_Pw_i16ReqPwrForHeat3 : Inport  Port=65  OutDataTypeStr=int16
  sTmSigProces_Te_s32CompDischarge3 : Inport  Port=66  OutDataTypeStr=single
  sTmSigProces_md_u16BlwCool3 : Inport  Port=67  OutDataTypeStr=uint16
  sTmSigProces_p_u16PHighSide3 : Inport  Port=68  OutDataTypeStr=uint16
  sTmSigProces_p_u16PLowSide3 : Inport  Port=69  OutDataTypeStr=uint16
  sTmIn_D_u8HeatPump3 : Inport  Port=70  OutDataTypeStr=uint8
  sTmIn_D_u8ElecDriveline3 : Inport  Port=71
  sTmSigProces_D_u8CarChrgMode3 : Inport  Port=72  OutDataTypeStr=uint8
  sTmSigProces_md_u16BlwHeat3 : Inport  Port=73  OutDataTypeStr=uint16
  sTmDiag_D_u8LoSidePFltSt3 : Inport  Port=74  OutDataTypeStr=uint8
  xTmComprCtrl_B_CompOnReqCompOn3 : Inport  Port=75  OutDataTypeStr=boolean
  Subsystem : Subsystem
  Subsystem1 : Subsystem
  Subsystem2 : Subsystem
  Subsystem3 : Subsystem
  rTmComprCtrl_n_u16CompRpmReqFilter : Outport  OutDataTypeStr=uint16
  xTmComprCtrl_B_KeepRpm : Outport  Port=2  OutDataTypeStr=boolean
  xFilter_B_ComprStop : Outport  Port=3  OutDataTypeStr=boolean
  sFilter_n_u16CompMaxRpm : Outport  Port=4  OutDataTypeStr=uint16
  rFilter_p_u16AcHiSideHiCut : Outport  Port=5  OutDataTypeStr=uint16
  rFilter_p_u16CmpLimitNormalP : Outport  Port=6  OutDataTypeStr=uint16
  rFilter_p_u16CmpLimitLowP : Outport  Port=7  OutDataTypeStr=uint16
  rFilter_p_u16CmpLimitMidP : Outport  Port=8  OutDataTypeStr=uint16
  rFilter_p_u16CmpLimitShutDownP : Outport  Port=9  OutDataTypeStr=uint16
  xTmComprCtrl_B_ReduceRpm : Outport  Port=10  OutDataTypeStr=boolean
  rTmComprCtrl_n_u16CompRpmReqFilter1 : Outport  Port=11  OutDataTypeStr=uint16
  xTmComprCtrl_B_KeepRpm1 : Outport  Port=12  OutDataTypeStr=boolean
  xFilter_B_ComprStop1 : Outport  Port=13  OutDataTypeStr=boolean
  sFilter_n_u16CompMaxRpm1 : Outport  Port=14  OutDataTypeStr=uint16
  rFilter_p_u16AcHiSideHiCut1 : Outport  Port=15  OutDataTypeStr=uint16
  rFilter_p_u16CmpLimitNormalP1 : Outport  Port=16  OutDataTypeStr=uint16
  rFilter_p_u16CmpLimitLowP1 : Outport  Port=17  OutDataTypeStr=uint16
  rFilter_p_u16CmpLimitMidP1 : Outport  Port=18  OutDataTypeStr=uint16
  rFilter_p_u16CmpLimitShutDownP1 : Outport  Port=19  OutDataTypeStr=uint16
  xTmComprCtrl_B_ReduceRpm1 : Outport  Port=20  OutDataTypeStr=boolean
  rTmComprCtrl_n_u16CompRpmReqFilter2 : Outport  Port=21  OutDataTypeStr=uint16
  xTmComprCtrl_B_KeepRpm2 : Outport  Port=22  OutDataTypeStr=boolean
  xFilter_B_ComprStop2 : Outport  Port=23  OutDataTypeStr=boolean
  sFilter_n_u16CompMaxRpm2 : Outport  Port=24  OutDataTypeStr=uint16
  rFilter_p_u16AcHiSideHiCut2 : Outport  Port=25  OutDataTypeStr=uint16
  rFilter_p_u16CmpLimitNormalP2 : Outport  Port=26  OutDataTypeStr=uint16
  rFilter_p_u16CmpLimitLowP2 : Outport  Port=27  OutDataTypeStr=uint16
  rFilter_p_u16CmpLimitMidP2 : Outport  Port=28  OutDataTypeStr=uint16
  rFilter_p_u16CmpLimitShutDownP2 : Outport  Port=29  OutDataTypeStr=uint16
  xTmComprCtrl_B_ReduceRpm2 : Outport  Port=30  OutDataTypeStr=boolean
  rTmComprCtrl_n_u16CompRpmReqFilter3 : Outport  Port=31  OutDataTypeStr=uint16
  xTmComprCtrl_B_KeepRpm3 : Outport  Port=32  OutDataTypeStr=boolean
  xFilter_B_ComprStop3 : Outport  Port=33  OutDataTypeStr=boolean
  sFilter_n_u16CompMaxRpm3 : Outport  Port=34  OutDataTypeStr=uint16
  rFilter_p_u16AcHiSideHiCut3 : Outport  Port=35  OutDataTypeStr=uint16
  rFilter_p_u16CmpLimitNormalP3 : Outport  Port=36  OutDataTypeStr=uint16
  rFilter_p_u16CmpLimitLowP3 : Outport  Port=37  OutDataTypeStr=uint16
  rFilter_p_u16CmpLimitMidP3 : Outport  Port=38  OutDataTypeStr=uint16
  rFilter_p_u16CmpLimitShutDownP3 : Outport  Port=39  OutDataTypeStr=uint16
  xTmComprCtrl_B_ReduceRpm3 : Outport  Port=40  OutDataTypeStr=boolean
  wires:
  Subsystem/7(rFilter_p_u16CmpLimitLowP) -> rFilter_p_u16CmpLimitLowP/1
  Subsystem/2(xTmComprCtrl_B_KeepRpm) -> xTmComprCtrl_B_KeepRpm/1
  Subsystem/8(rFilter_p_u16CmpLimitMidP) -> rFilter_p_u16CmpLimitMidP/1
  Subsystem/9(rFilter_p_u16CmpLimitShutDownP) -> rFilter_p_u16CmpLimitShutDownP/1
  Subsystem/6(rFilter_p_u16CmpLimitNormalP) -> rFilter_p_u16CmpLimitNormalP/1
  Subsystem/5(rFilter_p_u16AcHiSideHiCut) -> rFilter_p_u16AcHiSideHiCut/1
  Subsystem/3(xFilter_B_ComprStop) -> xFilter_B_ComprStop/1
  Subsystem/4(sFilter_n_u16CompMaxRpm) -> sFilter_n_u16CompMaxRpm/1
  sTmSigProces_D_u8CarChrgMode/1 -> Subsystem/18(sTmSigProces_D_u8CarChrgMode)
  sTmSigProces_md_u16BlwHeat/1 -> Subsystem/19(sTmSigProces_md_u16BlwHeat)
  sTmSigProces_p_u16PLowSide/1 -> Subsystem/15(sTmSigProces_p_u16PLowSide)
  sTmIn_D_u8HeatPump/1 -> Subsystem/16(sTmIn_D_u8HeatPump)
  sTmIn_D_u8ElecDriveline/1 -> Subsystem/17(sTmIn_D_u8ElecDriveline)
  sTmDiag_D_u8LoSidePFltSt/1 -> Subsystem/20(sTmDiag_D_u8LoSidePFltSt)
  sTmSigProces_Te_s32TAmb/1 -> Subsystem/6(sTmSigProces_Te_s32TAmb)
  sTmIn_n_s32ElacCmprActl/1 -> Subsystem/7(sTmIn_n_s32ElacCmprActl)
  sTmSigProces_Te_s32CompDischarge/1 -> Subsystem/12(sTmSigProces_Te_s32CompDischarge)
  sTmRefriModeMgr_D_u8HPCurMode/1 -> Subsystem/9(sTmRefriModeMgr_D_u8HPCurMode)
  sTmSigProces_Pw_i16ReqPwrForHeat/1 -> Subsystem/11(sTmSigProces_Pw_i16ReqPwrForHeat)
  sTmRefriModeMgr_D_u8HpFmCmd/1 -> Subsystem/10(sTmRefriModeMgr_D_u8HpFmCmd)
  sTmDiag_D_u8OutrCondOutTFltSt/1 -> Subsystem/5(sTmDiag_D_u8OutrCondOutTFltSt)
  sTmIn_v_s32VehSpdLgt/1 -> Subsystem/8(sTmIn_v_s32VehSpdLgt)
  sTmSigProces_md_u16BlwCool/1 -> Subsystem/13(sTmSigProces_md_u16BlwCool)
  sTmDiag_D_u8FanFltSt/1 -> Subsystem/3(sTmDiag_D_u8FanFltSt)
  sTmDiag_D_u8HiSidePFltSt/1 -> Subsystem/4(sTmDiag_D_u8HiSidePFltSt)
  xTmComprCtrl_B_CompOnReqCompOn/1 -> Subsystem/21(xTmComprCtrl_B_CompOnReqCompOn)
  sTmDiag_D_u8CmprDischrgTFltSt/1 -> Subsystem/2(sTmDiag_D_u8CmprDischrgTFltSt)
  rTmComprCtrl_n_u16CompRpmReqModeOut/1 -> Subsystem/1(rTmComprCtrl_n_u16CompRpmReqModeOut)
  Subsystem/1(rTmComprCtrl_n_u16CompRpmReqFilter) -> rTmComprCtrl_n_u16CompRpmReqFilter/1
  sTmSigProces_p_u16PHighSide/1 -> Subsystem/14(sTmSigProces_p_u16PHighSide)
  Subsystem/10(xTmComprCtrl_B_ReduceRpm) -> xTmComprCtrl_B_ReduceRpm/1
  Subsystem1/1(rTmComprCtrl_n_u16CompRpmReqFilter) -> rTmComprCtrl_n_u16CompRpmReqFilter1/1
  Subsystem1/10(xTmComprCtrl_B_ReduceRpm) -> xTmComprCtrl_B_ReduceRpm1/1
  rTmComprCtrl_n_u16CompRpmReqModeOut1/1 -> Subsystem1/1(rTmComprCtrl_n_u16CompRpmReqModeOut)
  sTmDiag_D_u8HiSidePFltSt1/1 -> Subsystem1/4(sTmDiag_D_u8HiSidePFltSt)
  sTmDiag_D_u8FanFltSt1/1 -> Subsystem1/3(sTmDiag_D_u8FanFltSt)
  Subsystem1/2(xTmComprCtrl_B_KeepRpm) -> xTmComprCtrl_B_KeepRpm1/1
  Subsystem1/7(rFilter_p_u16CmpLimitLowP) -> rFilter_p_u16CmpLimitLowP1/1
  sTmDiag_D_u8OutrCondOutTFltSt1/1 -> Subsystem1/5(sTmDiag_D_u8OutrCondOutTFltSt)
  sTmSigProces_Pw_i16ReqPwrForHeat1/1 -> Subsystem1/11(sTmSigProces_Pw_i16ReqPwrForHeat)
  sTmRefriModeMgr_D_u8HpFmCmd1/1 -> Subsystem1/10(sTmRefriModeMgr_D_u8HpFmCmd)
  sTmSigProces_Te_s32CompDischarge1/1 -> Subsystem1/12(sTmSigProces_Te_s32CompDischarge)
  sTmIn_n_s32ElacCmprActl1/1 -> Subsystem1/7(sTmIn_n_s32ElacCmprActl)
  sTmRefriModeMgr_D_u8HPCurMode1/1 -> Subsystem1/9(sTmRefriModeMgr_D_u8HPCurMode)
  sTmIn_v_s32VehSpdLgt1/1 -> Subsystem1/8(sTmIn_v_s32VehSpdLgt)
  Subsystem1/3(xFilter_B_ComprStop) -> xFilter_B_ComprStop1/1
  sTmSigProces_Te_s32TAmb1/1 -> Subsystem1/6(sTmSigProces_Te_s32TAmb)
  Subsystem1/5(rFilter_p_u16AcHiSideHiCut) -> rFilter_p_u16AcHiSideHiCut1/1
  sTmDiag_D_u8CmprDischrgTFltSt1/1 -> Subsystem1/2(sTmDiag_D_u8CmprDischrgTFltSt)
  Subsystem1/6(rFilter_p_u16CmpLimitNormalP) -> rFilter_p_u16CmpLimitNormalP1/1
  Subsystem1/4(sFilter_n_u16CompMaxRpm) -> sFilter_n_u16CompMaxRpm1/1
  Subsystem1/9(rFilter_p_u16CmpLimitShutDownP) -> rFilter_p_u16CmpLimitShutDownP1/1
  Subsystem1/8(rFilter_p_u16CmpLimitMidP) -> rFilter_p_u16CmpLimitMidP1/1
  Subsystem2/1(rTmComprCtrl_n_u16CompRpmReqFilter) -> rTmComprCtrl_n_u16CompRpmReqFilter2/1
  Subsystem2/10(xTmComprCtrl_B_ReduceRpm) -> xTmComprCtrl_B_ReduceRpm2/1
  sTmSigProces_p_u16PHighSide2/1 -> Subsystem2/14(sTmSigProces_p_u16PHighSide)
  rTmComprCtrl_n_u16CompRpmReqModeOut2/1 -> Subsystem2/1(rTmComprCtrl_n_u16CompRpmReqModeOut)
  sTmDiag_D_u8HiSidePFltSt2/1 -> Subsystem2/4(sTmDiag_D_u8HiSidePFltSt)
  sTmDiag_D_u8FanFltSt2/1 -> Subsystem2/3(sTmDiag_D_u8FanFltSt)
  Subsystem2/2(xTmComprCtrl_B_KeepRpm) -> xTmComprCtrl_B_KeepRpm2/1
  Subsystem2/7(rFilter_p_u16CmpLimitLowP) -> rFilter_p_u16CmpLimitLowP2/1
  sTmSigProces_md_u16BlwCool2/1 -> Subsystem2/13(sTmSigProces_md_u16BlwCool)
  sTmDiag_D_u8LoSidePFltSt2/1 -> Subsystem2/20(sTmDiag_D_u8LoSidePFltSt)
  sTmDiag_D_u8OutrCondOutTFltSt2/1 -> Subsystem2/5(sTmDiag_D_u8OutrCondOutTFltSt)
  xTmComprCtrl_B_CompOnReqCompOn2/1 -> Subsystem2/21(xTmComprCtrl_B_CompOnReqCompOn)
  sTmSigProces_Pw_i16ReqPwrForHeat2/1 -> Subsystem2/11(sTmSigProces_Pw_i16ReqPwrForHeat)
  sTmRefriModeMgr_D_u8HpFmCmd2/1 -> Subsystem2/10(sTmRefriModeMgr_D_u8HpFmCmd)
  sTmSigProces_Te_s32CompDischarge2/1 -> Subsystem2/12(sTmSigProces_Te_s32CompDischarge)
  sTmIn_n_s32ElacCmprActl2/1 -> Subsystem2/7(sTmIn_n_s32ElacCmprActl)
  sTmIn_D_u8HeatPump2/1 -> Subsystem2/16(sTmIn_D_u8HeatPump)
  sTmSigProces_p_u16PLowSide2/1 -> Subsystem2/15(sTmSigProces_p_u16PLowSide)
  sTmRefriModeMgr_D_u8HPCurMode2/1 -> Subsystem2/9(sTmRefriModeMgr_D_u8HPCurMode)
  sTmIn_v_s32VehSpdLgt2/1 -> Subsystem2/8(sTmIn_v_s32VehSpdLgt)
  sTmSigProces_D_u8CarChrgMode2/1 -> Subsystem2/18(sTmSigProces_D_u8CarChrgMode)
  Subsystem2/3(xFilter_B_ComprStop) -> xFilter_B_ComprStop2/1
  sTmSigProces_Te_s32TAmb2/1 -> Subsystem2/6(sTmSigProces_Te_s32TAmb)
  sTmSigProces_md_u16BlwHeat2/1 -> Subsystem2/19(sTmSigProces_md_u16BlwHeat)
  Subsystem2/5(rFilter_p_u16AcHiSideHiCut) -> rFilter_p_u16AcHiSideHiCut2/1
  sTmDiag_D_u8CmprDischrgTFltSt2/1 -> Subsystem2/2(sTmDiag_D_u8CmprDischrgTFltSt)
  Subsystem2/6(rFilter_p_u16CmpLimitNormalP) -> rFilter_p_u16CmpLimitNormalP2/1
  Subsystem2/4(sFilter_n_u16CompMaxRpm) -> sFilter_n_u16CompMaxRpm2/1
  sTmIn_D_u8ElecDriveline2/1 -> Subsystem2/17(sTmIn_D_u8ElecDriveline)
  Subsystem2/9(rFilter_p_u16CmpLimitShutDownP) -> rFilter_p_u16CmpLimitShutDownP2/1
  Subsystem2/8(rFilter_p_u16CmpLimitMidP) -> rFilter_p_u16CmpLimitMidP2/1
  Subsystem3/1(rTmComprCtrl_n_u16CompRpmReqFilter) -> rTmComprCtrl_n_u16CompRpmReqFilter3/1
  Subsystem3/10(xTmComprCtrl_B_ReduceRpm) -> xTmComprCtrl_B_ReduceRpm3/1
  sTmSigProces_p_u16PHighSide3/1 -> Subsystem3/14(sTmSigProces_p_u16PHighSide)
  rTmComprCtrl_n_u16CompRpmReqModeOut3/1 -> Subsystem3/1(rTmComprCtrl_n_u16CompRpmReqModeOut)
  sTmDiag_D_u8HiSidePFltSt3/1 -> Subsystem3/4(sTmDiag_D_u8HiSidePFltSt)
  sTmDiag_D_u8FanFltSt3/1 -> Subsystem3/3(sTmDiag_D_u8FanFltSt)
  Subsystem3/2(xTmComprCtrl_B_KeepRpm) -> xTmComprCtrl_B_KeepRpm3/1
  Subsystem3/7(rFilter_p_u16CmpLimitLowP) -> rFilter_p_u16CmpLimitLowP3/1
  sTmSigProces_md_u16BlwCool3/1 -> Subsystem3/13(sTmSigProces_md_u16BlwCool)
  sTmDiag_D_u8LoSidePFltSt3/1 -> Subsystem3/20(sTmDiag_D_u8LoSidePFltSt)
  sTmDiag_D_u8OutrCondOutTFltSt3/1 -> Subsystem3/5(sTmDiag_D_u8OutrCondOutTFltSt)
  xTmComprCtrl_B_CompOnReqCompOn3/1 -> Subsystem3/21(xTmComprCtrl_B_CompOnReqCompOn)
  sTmSigProces_Pw_i16ReqPwrForHeat3/1 -> Subsystem3/11(sTmSigProces_Pw_i16ReqPwrForHeat)
  sTmRefriModeMgr_D_u8HpFmCmd3/1 -> Subsystem3/10(sTmRefriModeMgr_D_u8HpFmCmd)
  sTmSigProces_Te_s32CompDischarge3/1 -> Subsystem3/12(sTmSigProces_Te_s32CompDischarge)
  sTmIn_n_s32ElacCmprActl3/1 -> Subsystem3/7(sTmIn_n_s32ElacCmprActl)
  sTmIn_D_u8HeatPump3/1 -> Subsystem3/16(sTmIn_D_u8HeatPump)
  sTmSigProces_p_u16PLowSide3/1 -> Subsystem3/15(sTmSigProces_p_u16PLowSide)
  sTmRefriModeMgr_D_u8HPCurMode3/1 -> Subsystem3/9(sTmRefriModeMgr_D_u8HPCurMode)
  sTmIn_v_s32VehSpdLgt3/1 -> Subsystem3/8(sTmIn_v_s32VehSpdLgt)
  sTmSigProces_D_u8CarChrgMode3/1 -> Subsystem3/18(sTmSigProces_D_u8CarChrgMode)
  Subsystem3/3(xFilter_B_ComprStop) -> xFilter_B_ComprStop3/1
  sTmSigProces_Te_s32TAmb3/1 -> Subsystem3/6(sTmSigProces_Te_s32TAmb)
  sTmSigProces_md_u16BlwHeat3/1 -> Subsystem3/19(sTmSigProces_md_u16BlwHeat)
  Subsystem3/5(rFilter_p_u16AcHiSideHiCut) -> rFilter_p_u16AcHiSideHiCut3/1
  sTmDiag_D_u8CmprDischrgTFltSt3/1 -> Subsystem3/2(sTmDiag_D_u8CmprDischrgTFltSt)
  Subsystem3/6(rFilter_p_u16CmpLimitNormalP) -> rFilter_p_u16CmpLimitNormalP3/1
  Subsystem3/4(sFilter_n_u16CompMaxRpm) -> sFilter_n_u16CompMaxRpm3/1
  sTmIn_D_u8ElecDriveline3/1 -> Subsystem3/17(sTmIn_D_u8ElecDriveline)
  Subsystem3/9(rFilter_p_u16CmpLimitShutDownP) -> rFilter_p_u16CmpLimitShutDownP3/1
  Subsystem3/8(rFilter_p_u16CmpLimitMidP) -> rFilter_p_u16CmpLimitMidP3/1

== system ScriptDemo/Change/changePortBlockPosAll/After1 ==
  rTmComprCtrl_n_u16CompRpmReqModeOut : Inport  OutDataTypeStr=uint16
  sTmDiag_D_u8CmprDischrgTFltSt : Inport  Port=2  OutDataTypeStr=uint8
  sTmDiag_D_u8FanFltSt : Inport  Port=3  OutDataTypeStr=uint8
  sTmDiag_D_u8HiSidePFltSt : Inport  Port=4  OutDataTypeStr=uint8
  sTmDiag_D_u8OutrCondOutTFltSt : Inport  Port=5  OutDataTypeStr=uint8
  sTmSigProces_Te_s32TAmb : Inport  Port=6  OutDataTypeStr=single
  sTmIn_n_s32ElacCmprActl : Inport  Port=7  OutDataTypeStr=single
  sTmIn_v_s32VehSpdLgt : Inport  Port=8  OutDataTypeStr=single
  sTmRefriModeMgr_D_u8HPCurMode : Inport  Port=9  OutDataTypeStr=uint8
  sTmRefriModeMgr_D_u8HpFmCmd : Inport  Port=10  OutDataTypeStr=uint8
  sTmSigProces_Pw_i16ReqPwrForHeat : Inport  Port=11  OutDataTypeStr=int16
  sTmSigProces_Te_s32CompDischarge : Inport  Port=12  OutDataTypeStr=single
  sTmSigProces_md_u16BlwCool : Inport  Port=13  OutDataTypeStr=uint16
  sTmSigProces_p_u16PHighSide : Inport  Port=14  OutDataTypeStr=uint16
  sTmSigProces_p_u16PLowSide : Inport  Port=15  OutDataTypeStr=uint16
  sTmIn_D_u8HeatPump : Inport  Port=16  OutDataTypeStr=uint8
  sTmIn_D_u8ElecDriveline : Inport  Port=17
  sTmSigProces_D_u8CarChrgMode : Inport  Port=18  OutDataTypeStr=uint8
  sTmSigProces_md_u16BlwHeat : Inport  Port=19  OutDataTypeStr=uint16
  sTmDiag_D_u8LoSidePFltSt : Inport  Port=20  OutDataTypeStr=uint8
  xTmComprCtrl_B_CompOnReqCompOn : Inport  Port=21  OutDataTypeStr=boolean
  rTmComprCtrl_n_u16CompRpmReqFilter : Outport  OutDataTypeStr=uint16
  xTmComprCtrl_B_KeepRpm : Outport  Port=2  OutDataTypeStr=boolean
  xFilter_B_ComprStop : Outport  Port=3  OutDataTypeStr=boolean
  sFilter_n_u16CompMaxRpm : Outport  Port=4  OutDataTypeStr=uint16
  rFilter_p_u16AcHiSideHiCut : Outport  Port=5  OutDataTypeStr=uint16
  rFilter_p_u16CmpLimitNormalP : Outport  Port=6  OutDataTypeStr=uint16
  rFilter_p_u16CmpLimitLowP : Outport  Port=7  OutDataTypeStr=uint16
  rFilter_p_u16CmpLimitMidP : Outport  Port=8  OutDataTypeStr=uint16
  rFilter_p_u16CmpLimitShutDownP : Outport  Port=9  OutDataTypeStr=uint16
  xTmComprCtrl_B_ReduceRpm : Outport  Port=10  OutDataTypeStr=boolean
  wires:
  [rTmComprCtrl_p_u16AcHiSideHiCut] -> rFilter_p_u16AcHiSideHiCut/1
  sTmRefriModeMgr_D_u8HpFmCmd/1 -> [sTmRefriModeMgr_D_u8HpFmCmd]
  sTmSigProces_p_u16PLowSide/1 -> [sTmSigProces_p_u16PLowSide]
  sTmSigProces_md_u16BlwHeat/1 -> [sTmSigProces_md_u16BlwHeat]
  sTmIn_n_s32ElacCmprActl/1 -> [sTmIn_n_s32ElacCmprActl]
  [xTmComprCtrl_B_ComprStop] -> xFilter_B_ComprStop/1
  [rTmComprCtrl_n_u16CompRpmReqCompOn] -> rTmComprCtrl_n_u16CompRpmReqFilter/1
  sTmDiag_D_u8OutrCondOutTFltSt/1 -> [sTmDiag_D_u8OutrCondOutTFltSt]
  sTmSigProces_md_u16BlwCool/1 -> [sTmSigProces_md_u16BlwCool]
  sTmDiag_D_u8LoSidePFltSt/1 -> [sTmDiag_D_u8LoSidePFltSt]
  sTmSigProces_p_u16PHighSide/1 -> [sTmSigProces_p_u16PHighSide]
  [rTmComprCtrl_p_u16CmpLimitLowP] -> rFilter_p_u16CmpLimitLowP/1
  sTmRefriModeMgr_D_u8HPCurMode/1 -> [sTmRefriModeMgr_D_u8HPCurMode]
  [rTmComprCtrl_p_u16CmpLimitMidP] -> rFilter_p_u16CmpLimitMidP/1
  [xTmComprCtrl_B_KeepRpm] -> xTmComprCtrl_B_KeepRpm/1
  [rTmComprCtrl_p_u16CmpLimitNormalP] -> rFilter_p_u16CmpLimitNormalP/1
  [rTmComprCtrl_p_u16CmpLimitShutDownP] -> rFilter_p_u16CmpLimitShutDownP/1
  sTmSigProces_Te_s32CompDischarge/1 -> [sTmSigProces_Te_s32CompDischarge]
  [xTmComprCtrl_B_ReduceRpm] -> xTmComprCtrl_B_ReduceRpm/1
  sTmIn_D_u8HeatPump/1 -> [sTmIn_D_u8HeatPump]
  sTmIn_v_s32VehSpdLgt/1 -> [sTmIn_v_s32VehSpdLgt]
  sTmIn_D_u8ElecDriveline/1 -> [sTmIn_D_u8ElecDriveline]
  [sTmComprCtrl_n_u16CompMaxRpm] -> sFilter_n_u16CompMaxRpm/1
  sTmDiag_D_u8HiSidePFltSt/1 -> [sTmDiag_D_u8HiSidePFltSt]
  sTmSigProces_D_u8CarChrgMode/1 -> [sTmSigProces_D_u8CarChrgMode]
  sTmSigProces_Te_s32TAmb/1 -> [sTmSigProces_Te_s32TAmb]
  rTmComprCtrl_n_u16CompRpmReqModeOut/1 -> [rTmComprCtrl_n_u16CompRpmReqModeOut]
  sTmDiag_D_u8CmprDischrgTFltSt/1 -> [sTmDiag_D_u8CmprDischrgTFltSt]
  sTmDiag_D_u8FanFltSt/1 -> [sTmDiag_D_u8FanFltSt]
  sTmSigProces_Pw_i16ReqPwrForHeat/1 -> [sTmSigProces_Pw_i16ReqPwrForHeat]
  xTmComprCtrl_B_CompOnReqCompOn/1 -> [xTmComprCtrl_B_CompOnReqCompOn]

== system ScriptDemo/Change/changePortBlockPosAll/Before ==
  rTmComprCtrl_n_u16CompRpmReqModeOut : Inport  OutDataTypeStr=uint16
  sTmDiag_D_u8CmprDischrgTFltSt : Inport  Port=2  OutDataTypeStr=uint8
  sTmDiag_D_u8FanFltSt : Inport  Port=3  OutDataTypeStr=uint8
  sTmDiag_D_u8HiSidePFltSt : Inport  Port=4  OutDataTypeStr=uint8
  sTmDiag_D_u8OutrCondOutTFltSt : Inport  Port=5  OutDataTypeStr=uint8
  sTmSigProces_Te_s32TAmb : Inport  Port=6  OutDataTypeStr=single
  sTmIn_n_s32ElacCmprActl : Inport  Port=7  OutDataTypeStr=single
  sTmIn_v_s32VehSpdLgt : Inport  Port=8  OutDataTypeStr=single
  sTmRefriModeMgr_D_u8HPCurMode : Inport  Port=9  OutDataTypeStr=uint8
  sTmRefriModeMgr_D_u8HpFmCmd : Inport  Port=10  OutDataTypeStr=uint8
  sTmSigProces_Pw_i16ReqPwrForHeat : Inport  Port=11  OutDataTypeStr=int16
  sTmSigProces_Te_s32CompDischarge : Inport  Port=12  OutDataTypeStr=single
  sTmSigProces_md_u16BlwCool : Inport  Port=13  OutDataTypeStr=uint16
  sTmSigProces_p_u16PHighSide : Inport  Port=14  OutDataTypeStr=uint16
  sTmSigProces_p_u16PLowSide : Inport  Port=15  OutDataTypeStr=uint16
  sTmIn_D_u8HeatPump : Inport  Port=16  OutDataTypeStr=uint8
  sTmIn_D_u8ElecDriveline : Inport  Port=17
  sTmSigProces_D_u8CarChrgMode : Inport  Port=18  OutDataTypeStr=uint8
  sTmSigProces_md_u16BlwHeat : Inport  Port=19  OutDataTypeStr=uint16
  sTmDiag_D_u8LoSidePFltSt : Inport  Port=20  OutDataTypeStr=uint8
  xTmComprCtrl_B_CompOnReqCompOn : Inport  Port=21  OutDataTypeStr=boolean
  sTmDiag_D_u8HiSidePNHPFltSt : Inport  Port=22  OutDataTypeStr=uint8
  rTmComprCtrl_n_u16CompRpmReqFilter : Outport  OutDataTypeStr=uint16
  xTmComprCtrl_B_KeepRpm : Outport  Port=2  OutDataTypeStr=boolean
  xFilter_B_ComprStop : Outport  Port=3  OutDataTypeStr=boolean
  sFilter_n_u16CompMaxRpm : Outport  Port=4  OutDataTypeStr=uint16
  rFilter_p_u16AcHiSideHiCut : Outport  Port=5  OutDataTypeStr=uint16
  rFilter_p_u16CmpLimitNormalP : Outport  Port=6  OutDataTypeStr=uint16
  rFilter_p_u16CmpLimitLowP : Outport  Port=7  OutDataTypeStr=uint16
  rFilter_p_u16CmpLimitMidP : Outport  Port=8  OutDataTypeStr=uint16
  rFilter_p_u16CmpLimitShutDownP : Outport  Port=9  OutDataTypeStr=uint16
  xTmComprCtrl_B_ReduceRpm : Outport  Port=10  OutDataTypeStr=boolean
  wires:
  sTmDiag_D_u8HiSidePFltSt/1 -> [sTmDiag_D_u8HiSidePFltSt]
  sTmRefriModeMgr_D_u8HpFmCmd/1 -> [sTmRefriModeMgr_D_u8HpFmCmd]
  sTmDiag_D_u8CmprDischrgTFltSt/1 -> [sTmDiag_D_u8CmprDischrgTFltSt]
  sTmSigProces_Te_s32TAmb/1 -> [sTmSigProces_Te_s32TAmb]
  rTmComprCtrl_n_u16CompRpmReqModeOut/1 -> [rTmComprCtrl_n_u16CompRpmReqModeOut]
  sTmDiag_D_u8OutrCondOutTFltSt/1 -> [sTmDiag_D_u8OutrCondOutTFltSt]
  sTmSigProces_p_u16PLowSide/1 -> [sTmSigProces_p_u16PLowSide]
  sTmSigProces_Pw_i16ReqPwrForHeat/1 -> [sTmSigProces_Pw_i16ReqPwrForHeat]
  sTmSigProces_D_u8CarChrgMode/1 -> [sTmSigProces_D_u8CarChrgMode]
  sTmSigProces_Te_s32CompDischarge/1 -> [sTmSigProces_Te_s32CompDischarge]
  sTmSigProces_p_u16PHighSide/1 -> [sTmSigProces_p_u16PHighSide]
  sTmDiag_D_u8HiSidePNHPFltSt/1 -> [sTmDiag_D_u8HiSidePNHPFltSt]
  sTmDiag_D_u8FanFltSt/1 -> [sTmDiag_D_u8FanFltSt]
  sTmSigProces_md_u16BlwHeat/1 -> [sTmSigProces_md_u16BlwHeat]
  xTmComprCtrl_B_CompOnReqCompOn/1 -> [xTmComprCtrl_B_CompOnReqCompOn]
  sTmRefriModeMgr_D_u8HPCurMode/1 -> [sTmRefriModeMgr_D_u8HPCurMode]
  sTmIn_v_s32VehSpdLgt/1 -> [sTmIn_v_s32VehSpdLgt]
  sTmIn_D_u8HeatPump/1 -> [sTmIn_D_u8HeatPump]
  sTmSigProces_md_u16BlwCool/1 -> [sTmSigProces_md_u16BlwCool]
  sTmDiag_D_u8LoSidePFltSt/1 -> [sTmDiag_D_u8LoSidePFltSt]
  sTmIn_n_s32ElacCmprActl/1 -> [sTmIn_n_s32ElacCmprActl]
  sTmIn_D_u8ElecDriveline/1 -> [sTmIn_D_u8ElecDriveline]
  [rTmComprCtrl_n_u16CompRpmReqCompOn] -> rTmComprCtrl_n_u16CompRpmReqFilter/1
  [xTmComprCtrl_B_KeepRpm] -> xTmComprCtrl_B_KeepRpm/1
  [sTmComprCtrl_n_u16CompMaxRpm] -> sFilter_n_u16CompMaxRpm/1
  [xTmComprCtrl_B_ComprStop] -> xFilter_B_ComprStop/1
  [rTmComprCtrl_p_u16AcHiSideHiCut] -> rFilter_p_u16AcHiSideHiCut/1
  [rTmComprCtrl_p_u16CmpLimitShutDownP] -> rFilter_p_u16CmpLimitShutDownP/1
  [rTmComprCtrl_p_u16CmpLimitNormalP] -> rFilter_p_u16CmpLimitNormalP/1
  [xTmComprCtrl_B_ReduceRpm] -> xTmComprCtrl_B_ReduceRpm/1
  [rTmComprCtrl_p_u16CmpLimitLowP] -> rFilter_p_u16CmpLimitLowP/1
  [rTmComprCtrl_p_u16CmpLimitMidP] -> rFilter_p_u16CmpLimitMidP/1

== system ScriptDemo/Change/changeSigType/Before ==
  rTmComprCtrl_n_s32CompRpmReqModeOut : Inport  OutDataTypeStr=uint16
  sTmDiag_D_u8CmprDischrgTFltSt : Inport  Port=2  OutDataTypeStr=uint8
  sTmDiag_D_u8FanFltSt : Inport  Port=3  OutDataTypeStr=uint8
  sTmDiag_D_u8HiSidePFltSt : Inport  Port=4  OutDataTypeStr=uint8
  sTmDiag_D_u8OutrCondOutTFltSt : Inport  Port=5  OutDataTypeStr=uint8
  sTmSigProces_Te_s32TAmb : Inport  Port=6  OutDataTypeStr=single
  sTmIn_n_s32ElacCmprActl : Inport  Port=7  OutDataTypeStr=single
  sTmIn_v_s32VehSpdLgt : Inport  Port=8  OutDataTypeStr=single
  sTmRefriModeMgr_D_u8HPCurMode : Inport  Port=9  OutDataTypeStr=uint8
  sTmRefriModeMgr_D_u8HpFmCmd : Inport  Port=10  OutDataTypeStr=uint8
  sTmSigProces_Pw_i16ReqPwrForHeat : Inport  Port=11  OutDataTypeStr=int16
  sTmSigProces_Te_s32CompDischarge : Inport  Port=12  OutDataTypeStr=single
  sTmSigProces_md_u16BlwCool : Inport  Port=13  OutDataTypeStr=uint16
  sTmSigProces_p_u16PHighSide : Inport  Port=14  OutDataTypeStr=uint16
  sTmSigProces_p_u16PLowSide : Inport  Port=15  OutDataTypeStr=uint16
  sTmIn_D_u8HeatPump : Inport  Port=16  OutDataTypeStr=uint8
  sTmIn_D_u8ElecDriveline : Inport  Port=17
  sTmSigProces_D_u8CarChrgMode : Inport  Port=18  OutDataTypeStr=uint8
  sTmSigProces_md_u16BlwHeat : Inport  Port=19  OutDataTypeStr=uint16
  sTmDiag_D_u8LoSidePFltSt : Inport  Port=20  OutDataTypeStr=uint8
  xTmComprCtrl_B_CompOnReqCompOn : Inport  Port=21  OutDataTypeStr=boolean
  sTmDiag_D_u8HiSidePNHPFltSt : Inport  Port=22  OutDataTypeStr=uint8
  rTmComprCtrl_n_u16CompRpmReqFilter : Outport  OutDataTypeStr=uint16
  xTmComprCtrl_B_KeepRpm : Outport  Port=2  OutDataTypeStr=boolean
  xFilter_B_ComprStop : Outport  Port=3  OutDataTypeStr=boolean
  sFilter_n_u16CompMaxRpm : Outport  Port=4  OutDataTypeStr=uint16
  rFilter_p_u16AcHiSideHiCut : Outport  Port=5  OutDataTypeStr=uint16
  rFilter_p_u16CmpLimitNormalP : Outport  Port=6  OutDataTypeStr=uint16
  rFilter_p_u16CmpLimitLowP : Outport  Port=7  OutDataTypeStr=uint16
  rFilter_p_u16CmpLimitMidP : Outport  Port=8  OutDataTypeStr=uint16
  rFilter_p_u16CmpLimitShutDownP : Outport  Port=9  OutDataTypeStr=uint16
  xTmComprCtrl_B_ReduceRpm : Outport  Port=10  OutDataTypeStr=boolean
  wires:
  sTmDiag_D_u8HiSidePFltSt/1 -> [sTmDiag_D_u8HiSidePFltSt]
  sTmRefriModeMgr_D_u8HpFmCmd/1 -> [sTmRefriModeMgr_D_u8HpFmCmd]
  sTmDiag_D_u8CmprDischrgTFltSt/1 -> [sTmDiag_D_u8CmprDischrgTFltSt]
  sTmSigProces_Te_s32TAmb/1 -> [sTmSigProces_Te_s32TAmb]
  rTmComprCtrl_n_s32CompRpmReqModeOut/1 -> [rTmComprCtrl_n_u16CompRpmReqModeOut]
  sTmDiag_D_u8OutrCondOutTFltSt/1 -> [sTmDiag_D_u8OutrCondOutTFltSt]
  sTmSigProces_p_u16PLowSide/1 -> [sTmSigProces_p_u16PLowSide]
  sTmSigProces_Pw_i16ReqPwrForHeat/1 -> [sTmSigProces_Pw_i16ReqPwrForHeat]
  sTmSigProces_D_u8CarChrgMode/1 -> [sTmSigProces_D_u8CarChrgMode]
  sTmSigProces_Te_s32CompDischarge/1 -> [sTmSigProces_Te_s32CompDischarge]
  sTmSigProces_p_u16PHighSide/1 -> [sTmSigProces_p_u16PHighSide]
  sTmDiag_D_u8HiSidePNHPFltSt/1 -> [sTmDiag_D_u8HiSidePNHPFltSt]
  sTmDiag_D_u8FanFltSt/1 -> [sTmDiag_D_u8FanFltSt]
  sTmSigProces_md_u16BlwHeat/1 -> [sTmSigProces_md_u16BlwHeat]
  xTmComprCtrl_B_CompOnReqCompOn/1 -> [xTmComprCtrl_B_CompOnReqCompOn]
  sTmRefriModeMgr_D_u8HPCurMode/1 -> [sTmRefriModeMgr_D_u8HPCurMode]
  sTmIn_v_s32VehSpdLgt/1 -> [sTmIn_v_s32VehSpdLgt]
  sTmIn_D_u8HeatPump/1 -> [sTmIn_D_u8HeatPump]
  sTmSigProces_md_u16BlwCool/1 -> [sTmSigProces_md_u16BlwCool]
  sTmDiag_D_u8LoSidePFltSt/1 -> [sTmDiag_D_u8LoSidePFltSt]
  sTmIn_n_s32ElacCmprActl/1 -> [sTmIn_n_s32ElacCmprActl]
  sTmIn_D_u8ElecDriveline/1 -> [sTmIn_D_u8ElecDriveline]
  [rTmComprCtrl_n_u16CompRpmReqCompOn] -> rTmComprCtrl_n_u16CompRpmReqFilter/1
  [xTmComprCtrl_B_KeepRpm] -> xTmComprCtrl_B_KeepRpm/1
  [sTmComprCtrl_n_u16CompMaxRpm] -> sFilter_n_u16CompMaxRpm/1
  [xTmComprCtrl_B_ComprStop] -> xFilter_B_ComprStop/1
  [rTmComprCtrl_p_u16AcHiSideHiCut] -> rFilter_p_u16AcHiSideHiCut/1
  [rTmComprCtrl_p_u16CmpLimitShutDownP] -> rFilter_p_u16CmpLimitShutDownP/1
  [rTmComprCtrl_p_u16CmpLimitNormalP] -> rFilter_p_u16CmpLimitNormalP/1
  [xTmComprCtrl_B_ReduceRpm] -> xTmComprCtrl_B_ReduceRpm/1
  [rTmComprCtrl_p_u16CmpLimitLowP] -> rFilter_p_u16CmpLimitLowP/1
  [rTmComprCtrl_p_u16CmpLimitMidP] -> rFilter_p_u16CmpLimitMidP/1
